simulink model "ooooooooooooooo"  (R2024b)
settings: Solver=VariableStepAuto  StartTime=0.0  StopTime=10.0  RelTol=1e-3
values from neighbouring files (symbols this model uses):
  A4 = horzcat([0;0;0;0], A4)    [stabilita_AS.m]
  AA = A - B * K    [stabilita_AS.m]
  B = [0; 0; k]    [stabilita_AS.m]
  BB = [0; B]    [stabilita_AS.m]
  K = acker(A, B, desired_poles)    [stabilita_AS.m]
  L_oss = (1/epsilon) * L0    [stabilita_AS.m]
settings Model: Creator=costa  LastModifiedBy=costa

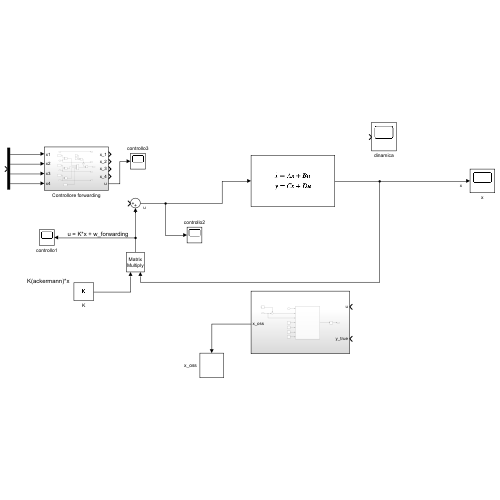
[thumbnail: Simulink's stored preview of the top-level diagram]
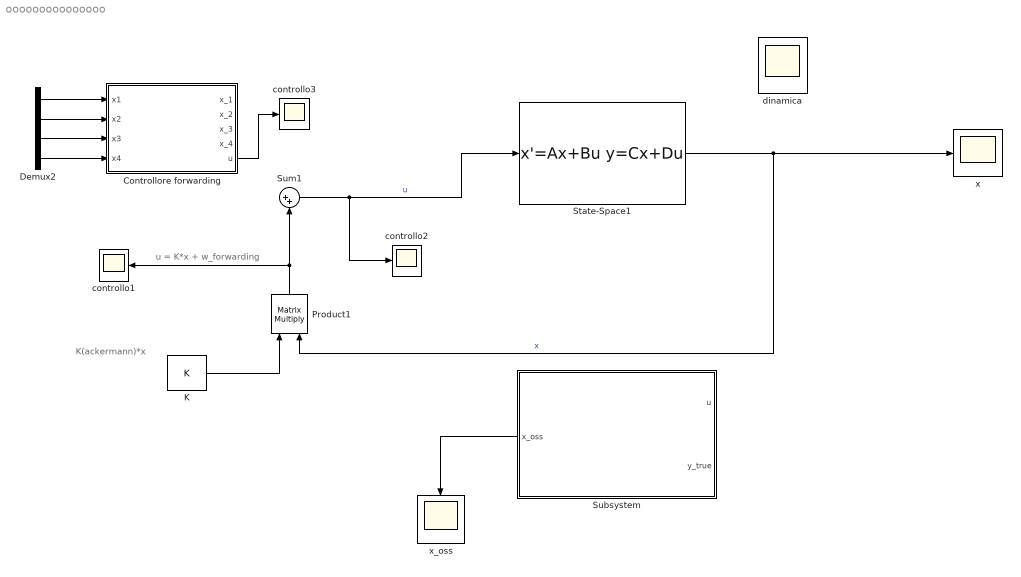
== system ooooooooooooooo ==
  note: K(ackermann)*x
  note: u = K*x + w_forwarding
  Controllore forwarding : Subsystem
  Demux2 : Demux
  K : Constant  Value=K  VectorParams1D=off
  Product1 : Product  Multiplication=Matrix(*)
  State-Space1 : StateSpace  A=AA  B=B  C=eye(4)  D=[0; 0; 0; 0]  InitialCondition=[1 0 1 0]
  Subsystem : Subsystem
  Sum1 : Sum  Inputs=|++
  controllo1 : Scope
  controllo2 : Scope
  controllo3 : Scope
  dinamica : Scope
  x : Scope
  x_oss : Scope
  wires:
  Controllore forwarding/5(u) -> controllo3/1
  Demux2/2 -> Controllore forwarding/2(x2)
  Demux2/4 -> Controllore forwarding/4(x4)
  Demux2/3 -> Controllore forwarding/3(x3)
  Subsystem/1(x_oss) -> x_oss/1
  Sum1/1 -> controllo2/1, State-Space1/1  "u"
  K/1 -> Product1/1
  Product1/1 -> controllo1/1, Sum1/2
  State-Space1/1 -> Product1/2, x/1  "x"
  Demux2/1 -> Controllore forwarding/1(x1)

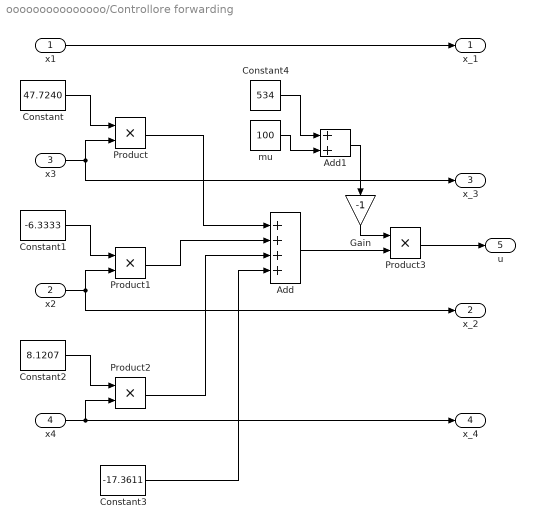
== system ooooooooooooooo/Controllore forwarding ==
  x1 : Inport
  x2 : Inport  Port=2
  x3 : Inport  Port=3
  x4 : Inport  Port=4
  Add : Sum  Inputs=++++
  Add1 : Sum
  Constant : Constant  Value=47.7240
  Constant1 : Constant  Value=-6.3333
  Constant2 : Constant  Value=8.1207
  Constant3 : Constant  Value=-17.3611
  Constant4 : Constant  Value=534
  Gain : Gain  Gain=-1
  Product{,1..3} (4 alike) : Product
  mu : Constant  Value=100
  x_1 : Outport
  x_2 : Outport  Port=2
  x_3 : Outport  Port=3
  x_4 : Outport  Port=4
  u : Outport  Port=5
  wires:
  x3/1 -> x_3/1, Product/2
  Constant/1 -> Product/1
  Constant1/1 -> Product1/1
  x2/1 -> Product1/2, x_2/1
  Constant2/1 -> Product2/1
  x4/1 -> x_4/1, Product2/2
  Product/1 -> Add/1
  Product1/1 -> Add/2
  Product2/1 -> Add/3
  Constant3/1 -> Add/4
  Add/1 -> Product3/2
  Product3/1 -> u/1
  x1/1 -> x_1/1
  Constant4/1 -> Add1/1
  mu/1 -> Add1/2
  Add1/1 -> Gain/1
  Gain/1 -> Product3/1

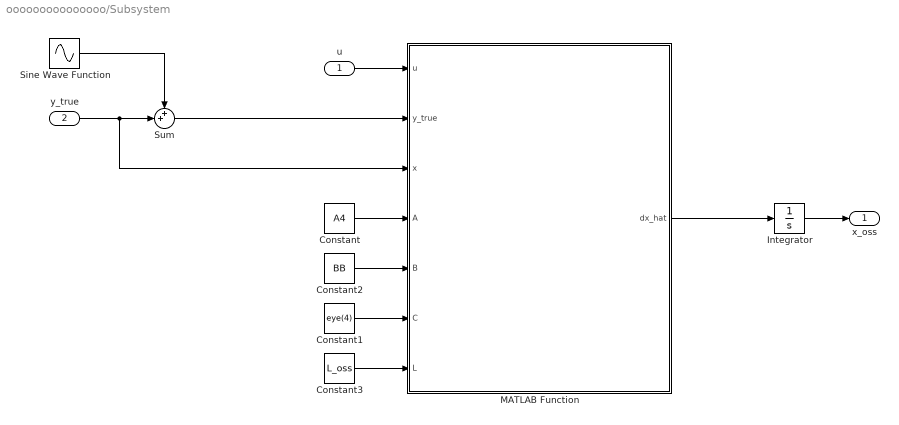
== system ooooooooooooooo/Subsystem ==
  u : Inport
  y_true : Inport  Port=2
  Constant : Constant  Value=A4  VectorParams1D=off
  Constant1 : Constant  Value=eye(4)
  Constant2 : Constant  Value=BB
  Constant3 : Constant  Value=L_oss  VectorParams1D=off
  Integrator : Integrator
  MATLAB Function : MATLAB Function  TreatAsAtomicUnit=on
  Sine Wave Function : Sin  TimeSource=Use external signal  Amplitude=0.1  Frequency=2*pi*50  SampleTime=0
  Sum : Sum  Inputs=++|
  x_oss : Outport
  wires:
  u/1 -> MATLAB Function/1(u)
  MATLAB Function/1(dx_hat) -> Integrator/1
  y_true/1 -> MATLAB Function/3(x), Sum/2
  Integrator/1 -> x_oss/1
  Constant1/1 -> MATLAB Function/6(C)
  Constant2/1 -> MATLAB Function/5(B)
  Constant/1 -> MATLAB Function/4(A)
  Constant3/1 -> MATLAB Function/7(L)
  Sum/1 -> MATLAB Function/2(y_true)
  Sine Wave Function/1 -> Sum/1

== matlab function ooooooooooooooo/Subsystem/MATLAB Function ==
  data: u input; dx_hat output; y_true input; x input; A input; B input; C input; L input
function dx_hat = fcn(u, y_true, x, A, B, C, L)
    dx_hat = A*x + B*u + L*(y_true-C*x);
end
